simulink library "seriallib"  (Simulink 5.0)
values from neighbouring files (symbols this model uses):
  count = count + 1    (= 5)    [mdecodestate.m]
undefined symbols (not defined in the file or in its folder): mbaseserialmask, mmodemcontrol, mquamask, mrs232
libraries: xpclib x193, vxlib x36, simulink x4
(part 3 of 3)

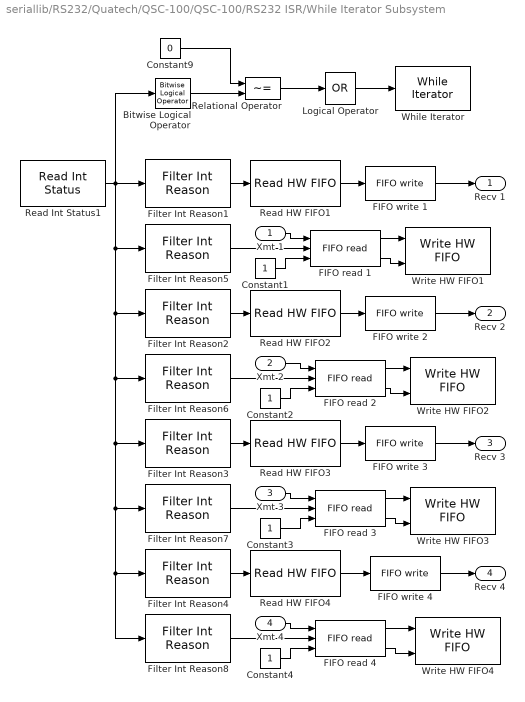
== system seriallib/RS232/Quatech/QSC-100/QSC-100/RS232 ISR/While Iterator Subsystem ==
  Xmt 1 : Inport
  Xmt 2 : Inport  Port=2
  Xmt 3 : Inport  Port=3
  Xmt 4 : Inport  Port=4
  Bitwise Logical Operator : simulink/Math Operations/Bitwise Logical Operator  Operator=AND  Operand2='FF'
  Constant{1..4} (4 alike) : Constant  ShowAdditionalParam=on  OutDataTypeMode=uint32
  Constant9 : Constant  Value=0  ShowAdditionalParam=on  OutDataTypeMode=uint32
  FIFO read {1..4} (4 alike) : xpclib/RS232/FIFO read   maxsize=60  minsize=1  usedelimiter=off  delimiter=13  outputtype=count+32 bit uint  enable=on  enableout=on  sampletime=-1
  FIFO write {1..4} (4 alike) : xpclib/RS232/FIFO write   size=1024  inputtype=count+32 bit uint  present=off  sampletime=-1
  Filter Int Reason1 : xpclib/RS232/Quatech/QSC-100/QSC-100 Internal  blocks/Filter Int Reason  port=1  value=Receive data
  Filter Int Reason2 : xpclib/RS232/Quatech/QSC-100/QSC-100 Internal  blocks/Filter Int Reason  port=2  value=Receive data
  Filter Int Reason3 : xpclib/RS232/Quatech/QSC-100/QSC-100 Internal  blocks/Filter Int Reason  port=3  value=Receive data
  Filter Int Reason4 : xpclib/RS232/Quatech/QSC-100/QSC-100 Internal  blocks/Filter Int Reason  port=4  value=Receive data
  Filter Int Reason5 : xpclib/RS232/Quatech/QSC-100/QSC-100 Internal  blocks/Filter Int Reason  port=1  value=Transmitter empty
  Filter Int Reason6 : xpclib/RS232/Quatech/QSC-100/QSC-100 Internal  blocks/Filter Int Reason  port=2  value=Transmitter empty
  Filter Int Reason7 : xpclib/RS232/Quatech/QSC-100/QSC-100 Internal  blocks/Filter Int Reason  port=3  value=Transmitter empty
  Filter Int Reason8 : xpclib/RS232/Quatech/QSC-100/QSC-100 Internal  blocks/Filter Int Reason  port=4  value=Transmitter empty
  Logical Operator : Logic  Operator=OR  Inputs=1  AllPortsSameDT=off
  Read HW FIFO1 : xpclib/RS232/Quatech/QSC-100/QSC-100 Internal  blocks/Read HW FIFO  port=1  flush=on  slot=subslot
  Read HW FIFO2 : xpclib/RS232/Quatech/QSC-100/QSC-100 Internal  blocks/Read HW FIFO  port=2  flush=on  slot=subslot
  Read HW FIFO3 : xpclib/RS232/Quatech/QSC-100/QSC-100 Internal  blocks/Read HW FIFO  port=3  flush=on  slot=subslot
  Read HW FIFO4 : xpclib/RS232/Quatech/QSC-100/QSC-100 Internal  blocks/Read HW FIFO  port=4  flush=on  slot=subslot
  Read Int Status1 : xpclib/RS232/Quatech/QSC-100/QSC-100 Internal  blocks/Read Int Status  slot=subslot
  Relational Operator : RelationalOperator  Operator=~=
  While Iterator : WhileIterator  MaxIters=65  WhileBlockType=do-while
  Write HW FIFO1 : xpclib/RS232/Quatech/QSC-100/QSC-100 Internal  blocks/Write HW FIFO  port=1  slot=subslot
  Write HW FIFO2 : xpclib/RS232/Quatech/QSC-100/QSC-100 Internal  blocks/Write HW FIFO  port=2  slot=subslot
  Write HW FIFO3 : xpclib/RS232/Quatech/QSC-100/QSC-100 Internal  blocks/Write HW FIFO  port=3  slot=subslot
  Write HW FIFO4 : xpclib/RS232/Quatech/QSC-100/QSC-100 Internal  blocks/Write HW FIFO  port=4  slot=subslot
  Recv 1 : Outport
  Recv 2 : Outport  Port=2
  Recv 3 : Outport  Port=3
  Recv 4 : Outport  Port=4
  wires:
  Constant9/1 -> Relational Operator/1
  Bitwise Logical Operator/1 -> Relational Operator/2
  Relational Operator/1 -> Logical Operator/1
  Logical Operator/1 -> While Iterator/1
  Constant4/1 -> FIFO read 4/3
  Constant3/1 -> FIFO read 3/3
  Constant2/1 -> FIFO read 2/3
  Constant1/1 -> FIFO read 1/3
  FIFO read 1/2 -> Write HW FIFO1/2
  FIFO read 1/1 -> Write HW FIFO1/1
  FIFO read 2/2 -> Write HW FIFO2/2
  FIFO read 2/1 -> Write HW FIFO2/1
  FIFO read 3/2 -> Write HW FIFO3/2
  FIFO read 3/1 -> Write HW FIFO3/1
  FIFO read 4/2 -> Write HW FIFO4/2
  FIFO read 4/1 -> Write HW FIFO4/1
  Read Int Status1/1 -> Bitwise Logical Operator/1, Filter Int Reason4/1, Filter Int Reason8/1, Filter Int Reason7/1, Filter Int Reason3/1, Filter Int Reason6/1, Filter Int Reason2/1, Filter Int Reason5/1, Filter Int Reason1/1
  Filter Int Reason1/1 -> Read HW FIFO1/1
  FIFO write 1/1 -> Recv 1/1
  Read HW FIFO1/1 -> FIFO write 1/1
  Filter Int Reason5/1 -> FIFO read 1/2
  Xmt 1/1 -> FIFO read 1/1
  Filter Int Reason2/1 -> Read HW FIFO2/1
  FIFO write 2/1 -> Recv 2/1
  Read HW FIFO2/1 -> FIFO write 2/1
  Filter Int Reason6/1 -> FIFO read 2/2
  Xmt 2/1 -> FIFO read 2/1
  Filter Int Reason3/1 -> Read HW FIFO3/1
  FIFO write 3/1 -> Recv 3/1
  Read HW FIFO3/1 -> FIFO write 3/1
  Filter Int Reason7/1 -> FIFO read 3/2
  Xmt 3/1 -> FIFO read 3/1
  Filter Int Reason4/1 -> Read HW FIFO4/1
  FIFO write 4/1 -> Recv 4/1
  Read HW FIFO4/1 -> FIFO write 4/1
  Filter Int Reason8/1 -> FIFO read 4/2
  Xmt 4/1 -> FIFO read 4/1

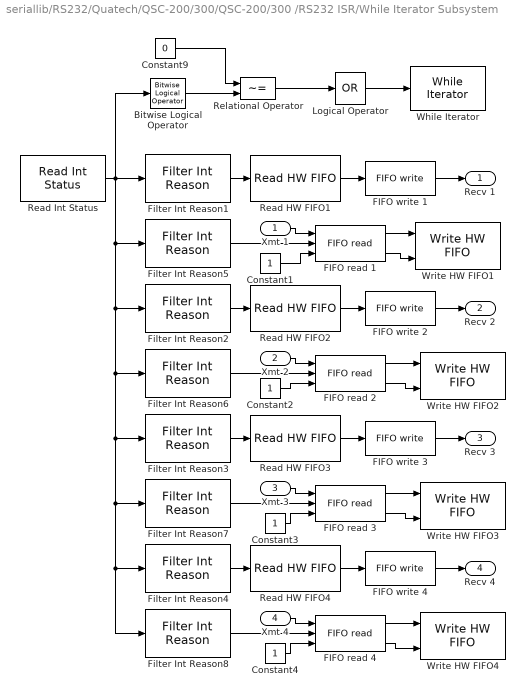
== system seriallib/RS232/Quatech/QSC-200/300/QSC-200/300 /RS232 ISR/While Iterator Subsystem ==
  Xmt 1 : Inport
  Xmt 2 : Inport  Port=2
  Xmt 3 : Inport  Port=3
  Xmt 4 : Inport  Port=4
  Bitwise Logical Operator : simulink/Math Operations/Bitwise Logical Operator  Operator=AND  Operand2='FF'
  Constant{1..4} (4 alike) : Constant  ShowAdditionalParam=on  OutDataTypeMode=uint32
  Constant9 : Constant  Value=0  ShowAdditionalParam=on  OutDataTypeMode=uint32
  FIFO read {1..4} (4 alike) : xpclib/RS232/FIFO read   maxsize=60  minsize=1  usedelimiter=off  delimiter=13  outputtype=count+32 bit uint  enable=on  enableout=on  sampletime=-1
  FIFO write {1..4} (4 alike) : xpclib/RS232/FIFO write   size=1024  inputtype=count+32 bit uint  present=off  sampletime=-1
  Filter Int Reason1 : xpclib/RS232/Quatech/QSC-200//300/QSC-200//300 Internal  blocks1/Filter Int Reason  port=1  value=Receive data
  Filter Int Reason2 : xpclib/RS232/Quatech/QSC-200//300/QSC-200//300 Internal  blocks1/Filter Int Reason  port=2  value=Receive data
  Filter Int Reason3 : xpclib/RS232/Quatech/QSC-200//300/QSC-200//300 Internal  blocks1/Filter Int Reason  port=3  value=Receive data
  Filter Int Reason4 : xpclib/RS232/Quatech/QSC-200//300/QSC-200//300 Internal  blocks1/Filter Int Reason  port=4  value=Receive data
  Filter Int Reason5 : xpclib/RS232/Quatech/QSC-200//300/QSC-200//300 Internal  blocks1/Filter Int Reason  port=1  value=Transmitter empty
  Filter Int Reason6 : xpclib/RS232/Quatech/QSC-200//300/QSC-200//300 Internal  blocks1/Filter Int Reason  port=2  value=Transmitter empty
  Filter Int Reason7 : xpclib/RS232/Quatech/QSC-200//300/QSC-200//300 Internal  blocks1/Filter Int Reason  port=3  value=Transmitter empty
  Filter Int Reason8 : xpclib/RS232/Quatech/QSC-200//300/QSC-200//300 Internal  blocks1/Filter Int Reason  port=4  value=Transmitter empty
  Logical Operator : Logic  Operator=OR  Inputs=1  AllPortsSameDT=off
  Read HW FIFO1 : xpclib/RS232/Quatech/QSC-200//300/QSC-200//300 Internal  blocks1/Read HW FIFO  port=1  flush=on  slot=subslot
  Read HW FIFO2 : xpclib/RS232/Quatech/QSC-200//300/QSC-200//300 Internal  blocks1/Read HW FIFO  port=2  flush=on  slot=subslot
  Read HW FIFO3 : xpclib/RS232/Quatech/QSC-200//300/QSC-200//300 Internal  blocks1/Read HW FIFO  port=3  flush=on  slot=subslot
  Read HW FIFO4 : xpclib/RS232/Quatech/QSC-200//300/QSC-200//300 Internal  blocks1/Read HW FIFO  port=4  flush=on  slot=subslot
  Read Int Status : xpclib/RS232/Quatech/QSC-200//300/QSC-200//300 Internal  blocks1/Read Int Status  slot=subslot
  Relational Operator : RelationalOperator  Operator=~=
  While Iterator : WhileIterator  MaxIters=65  WhileBlockType=do-while
  Write HW FIFO1 : xpclib/RS232/Quatech/QSC-200//300/QSC-200//300 Internal  blocks1/Write HW FIFO  port=1  onxmt=None  slot=subslot
  Write HW FIFO2 : xpclib/RS232/Quatech/QSC-200//300/QSC-200//300 Internal  blocks1/Write HW FIFO  port=2  onxmt=None  slot=subslot
  Write HW FIFO3 : xpclib/RS232/Quatech/QSC-200//300/QSC-200//300 Internal  blocks1/Write HW FIFO  port=3  onxmt=None  slot=subslot
  Write HW FIFO4 : xpclib/RS232/Quatech/QSC-200//300/QSC-200//300 Internal  blocks1/Write HW FIFO  port=4  onxmt=None  slot=subslot
  Recv 1 : Outport
  Recv 2 : Outport  Port=2
  Recv 3 : Outport  Port=3
  Recv 4 : Outport  Port=4
  wires:
  Constant9/1 -> Relational Operator/1
  Bitwise Logical Operator/1 -> Relational Operator/2
  Relational Operator/1 -> Logical Operator/1
  Logical Operator/1 -> While Iterator/1
  Constant4/1 -> FIFO read 4/3
  Constant3/1 -> FIFO read 3/3
  Constant2/1 -> FIFO read 2/3
  Constant1/1 -> FIFO read 1/3
  FIFO read 4/2 -> Write HW FIFO4/2
  FIFO read 2/2 -> Write HW FIFO2/2
  FIFO read 1/2 -> Write HW FIFO1/2
  FIFO read 1/1 -> Write HW FIFO1/1
  FIFO read 2/1 -> Write HW FIFO2/1
  FIFO read 3/2 -> Write HW FIFO3/2
  FIFO read 3/1 -> Write HW FIFO3/1
  FIFO read 4/1 -> Write HW FIFO4/1
  Xmt 4/1 -> FIFO read 4/1
  Filter Int Reason8/1 -> FIFO read 4/2
  Read HW FIFO4/1 -> FIFO write 4/1
  FIFO write 4/1 -> Recv 4/1
  Filter Int Reason4/1 -> Read HW FIFO4/1
  Xmt 3/1 -> FIFO read 3/1
  Filter Int Reason7/1 -> FIFO read 3/2
  Read HW FIFO3/1 -> FIFO write 3/1
  FIFO write 3/1 -> Recv 3/1
  Filter Int Reason3/1 -> Read HW FIFO3/1
  Xmt 2/1 -> FIFO read 2/1
  Filter Int Reason6/1 -> FIFO read 2/2
  Read HW FIFO2/1 -> FIFO write 2/1
  FIFO write 2/1 -> Recv 2/1
  Filter Int Reason2/1 -> Read HW FIFO2/1
  Xmt 1/1 -> FIFO read 1/1
  Filter Int Reason5/1 -> FIFO read 1/2
  Read HW FIFO1/1 -> FIFO write 1/1
  FIFO write 1/1 -> Recv 1/1
  Filter Int Reason1/1 -> Read HW FIFO1/1
  Read Int Status/1 -> Bitwise Logical Operator/1, Filter Int Reason4/1, Filter Int Reason8/1, Filter Int Reason7/1, Filter Int Reason3/1, Filter Int Reason6/1, Filter Int Reason2/1, Filter Int Reason5/1, Filter Int Reason1/1
